simulink model "Simulink_Demo"  (Simulink 8.3)
settings: Solver=ode3  StartTime=0.0  StopTime=10  FixedStep=0.01  RelTol=1e-3
values from neighbouring files (symbols this model uses):
  denK = [1 10 25 0]    [RongKutta.m]
  numK = [115]    [RongKutta.m]
undefined symbols (not defined in the file or in its folder): A, B, C, D, den, num
settings Model: Creator=李广文  LastModifiedBy=李广文
settings DataIOCC: SignalLoggingSaveFormat=Dataset
settings DebuggingCC: UnderspecifiedInitializationDetection=Simplified  StateNameClashWarn=none
settings GRTTargetCC: CombineOutputUpdateFcns=on  GRTInterface=off

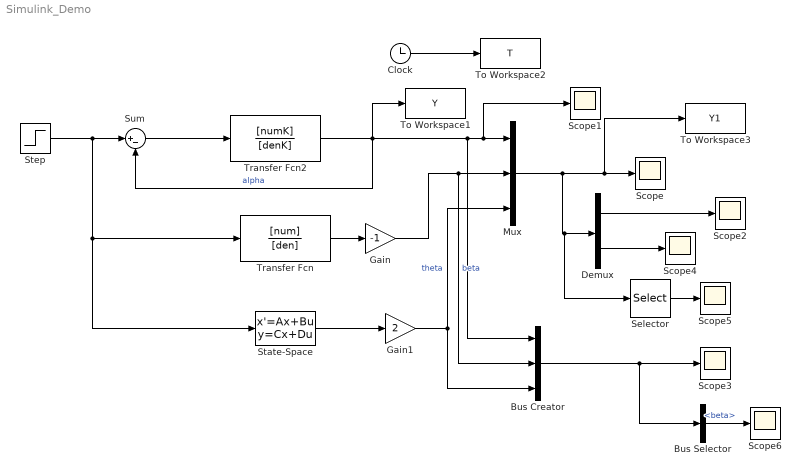
== system Simulink_Demo ==
  Bus Creator : BusCreator  Inputs=3
  Bus Selector : BusSelector  OutputSignals=beta
  Clock : Clock
  Demux : Demux  Outputs=2
  Gain : Gain  Gain=-1
  Gain1 : Gain  Gain=2
  Mux : Mux  Inputs=3
  Scope{,1..6} (7 alike) : Scope
      Scope2 settings: SaveName=ScopeData2
      Scope3 settings: SaveName=ScopeData3
      Scope4 settings: SaveName=ScopeData4
      Scope5 settings: SaveName=ScopeData5
      Scope6 settings: SaveName=ScopeData6
  Selector : Selector  InputPortWidth=3  Indices=[2 3]
  State-Space : StateSpace  A=A  B=B  C=C  D=D  X0=[0 0 0]
  Step : Step  Time=0  SampleTime=0
  Sum : Sum  Inputs=|+-
  To Workspace1 : ToWorkspace  VariableName=Y  SampleTime=-1
  To Workspace2 : ToWorkspace  VariableName=T  SampleTime=-1
  To Workspace3 : ToWorkspace  VariableName=Y1  SampleTime=-1
  Transfer Fcn : TransferFcn  Numerator=[num]  Denominator=[den]
  Transfer Fcn2 : TransferFcn  Numerator=[numK]  Denominator=[denK]
  wires:
  Step/1 -> State-Space/1, Transfer Fcn/1, Sum/1
  Sum/1 -> Transfer Fcn2/1
  Transfer Fcn2/1 -> Bus Creator/1, Scope1/1, Mux/1, To Workspace1/1, Sum/2  "alpha"
  Transfer Fcn/1 -> Gain/1
  State-Space/1 -> Gain1/1
  Mux/1 -> Selector/1, Demux/1, To Workspace3/1, Scope/1
  Clock/1 -> To Workspace2/1
  Gain/1 -> Bus Creator/2, Mux/2  "beta"
  Gain1/1 -> Bus Creator/3, Mux/3  "theta"
  Demux/1 -> Scope2/1
  Demux/2 -> Scope4/1
  Selector/1 -> Scope5/1
  Bus Creator/1 -> Bus Selector/1, Scope3/1
  Bus Selector/1 -> Scope6/1  "<beta>"
